simulink model "statespaceExSimulink2Observer"  (R2023b)
settings: Solver=VariableStepAuto  StartTime=0.0  StopTime=10.0  RelTol=1e-3
undefined symbols (not defined in the file): A, B, C, K, L
settings Model: Creator=klysm  LastModifiedBy=klysm

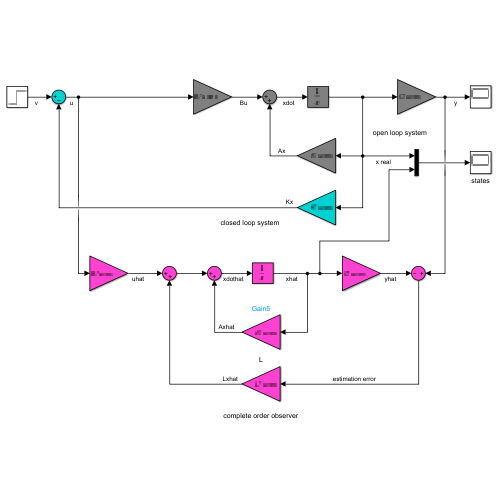
[thumbnail: Simulink's stored preview of the top-level diagram]
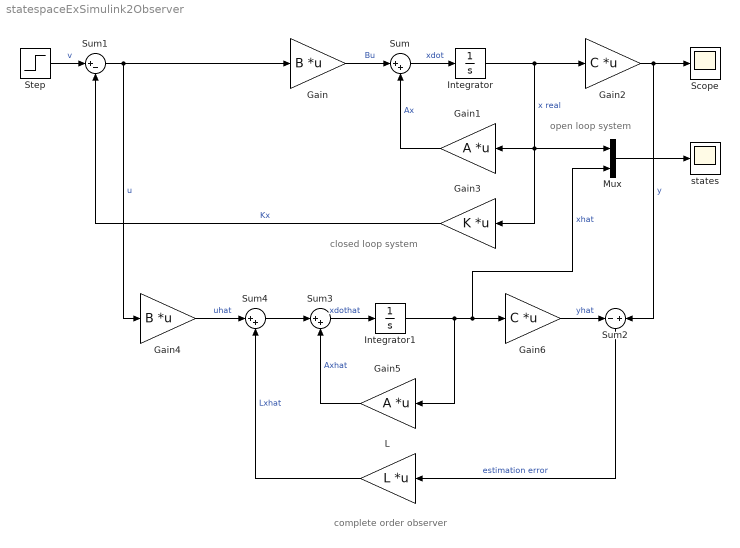
== system statespaceExSimulink2Observer ==
  note: open loop system
  note: closed loop system
  note: complete order observer
  Gain : Gain  Gain=B  Multiplication=Matrix(K*u) (u vector)
  Gain1 : Gain  Gain=A  Multiplication=Matrix(K*u) (u vector)
  Gain2 : Gain  Gain=C  Multiplication=Matrix(K*u) (u vector)
  Gain3 : Gain  Gain=K  Multiplication=Matrix(K*u) (u vector)
  Gain4 : Gain  Gain=B  Multiplication=Matrix(K*u) (u vector)
  Gain5 : Gain  Gain=A  Multiplication=Matrix(K*u) (u vector)
  Gain6 : Gain  Gain=C  Multiplication=Matrix(K*u) (u vector)
  Integrator : Integrator
  Integrator1 : Integrator
  L : Gain  Gain=L  Multiplication=Matrix(K*u) (u vector)
  Mux : Mux  Inputs=2
  Scope : Scope
  Step : Step  SampleTime=0
  Sum : Sum  Inputs=|++
  Sum1 : Sum  Inputs=|+-
  Sum2 : Sum  Inputs=-|+
  Sum3 : Sum  Inputs=|++
  Sum4 : Sum  Inputs=|++
  states : Scope
  wires:
  Sum/1 -> Integrator/1  "xdot"
  Gain1/1 -> Sum/2  "Ax"
  Gain/1 -> Sum/1  "Bu"
  Integrator/1 -> Gain2/1, Mux/1, Gain3/1, Gain1/1  "x real"
  Gain2/1 -> Sum2/2, Scope/1  "y"
  Sum1/1 -> Gain4/1, Gain/1  "u"
  Gain3/1 -> Sum1/2  "Kx"
  Step/1 -> Sum1/1  "v"
  Integrator1/1 -> Mux/2, Gain6/1, Gain5/1  "xhat"
  Gain5/1 -> Sum3/2  "Axhat"
  Sum3/1 -> Integrator1/1  "xdothat"
  Gain6/1 -> Sum2/1  "yhat"
  Sum2/1 -> L/1  "estimation error"
  Gain4/1 -> Sum4/1  "uhat"
  Sum4/1 -> Sum3/1
  L/1 -> Sum4/2  "Lxhat"
  Mux/1 -> states/1
